simulink model "project1_Harrington_and_Mckeon"  (R2025a)
settings: Solver=VariableStepAuto  StartTime=0.0  StopTime=30  RelTol=1e-3
model workspace (MAT data in the model file):
  A = 972
  M1 = 300
  M2 = 75
  g = 1.62
  k = 9000
  mu = 0.2
undefined symbols (not defined in the file): pulse
libraries: simulink x1
settings Model: Creator=brendan  LastModifiedBy=brendanharrington

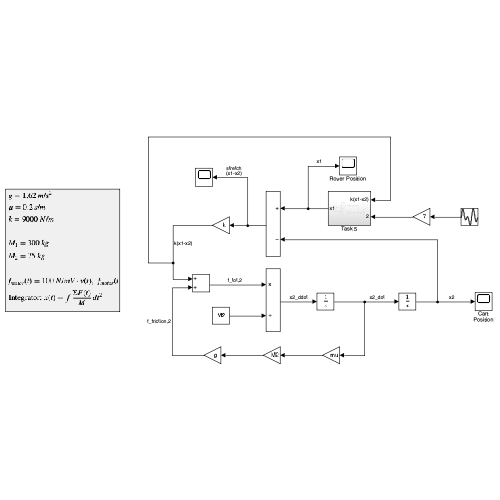
[thumbnail: Simulink's stored preview of the top-level diagram]
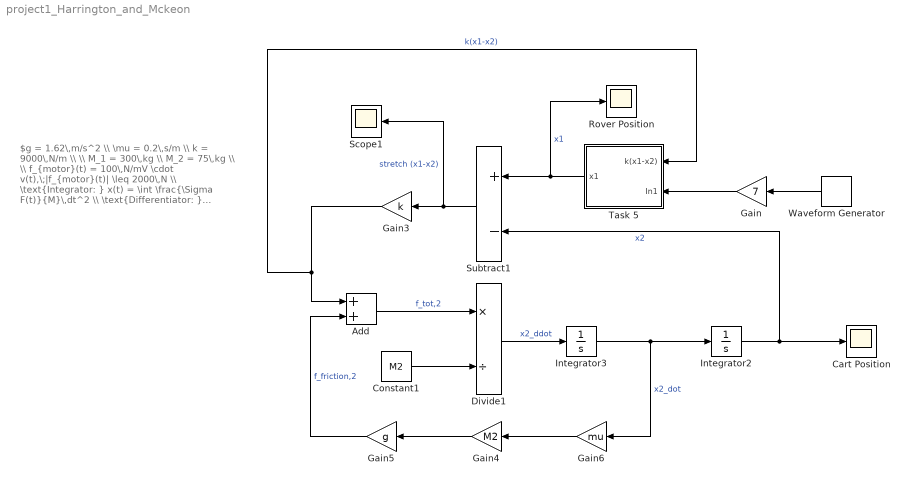
== system project1_Harrington_and_Mckeon ==
  note: $g = 1.62\,m/s^2 \\ \mu = 0.2\,s/m \\ k = 9000\,N/m \\ \\ M_1 = 300\,kg \\ M_2 = 75\,kg \\ \\ f_{motor}(t) = 100\,N/mV \cdot v(t),\;|f_{motor}(t)| \leq 2000\,N \\ \text{Integrator: } x(t) = \int \frac{\Sigma F(t)}{M}\,dt^2 \\ \text{Differentiator: } f_{friction}(t) = -\mu M g\,\dot{x}(t) \\ \\ \frac{X_1(s)}{F_{motor}(s)} = \frac{1}{M_1(s^2+\mu g s)}$
  Add : Sum
  Cart Position : Scope
      settings: ActiveDisplayYMinimum=-12.04250247875151  ActiveDisplayYMaximum=108.38252230876363  DataLoggingVariableName=ScopeData4
  Constant1 : Constant  Value=M2
  Divide1 : Product  Inputs=*/
  Gain : Gain  Gain=7
  Gain3 : Gain  Gain=k
  Gain4 : Gain  Gain=M2
  Gain5 : Gain  Gain=g
  Gain6 : Gain  Gain=mu
  Integrator2 : Integrator
  Integrator3 : Integrator
  Rover Position : Scope
      settings: ActiveDisplayYMinimum=-34.346909890801307  ActiveDisplayYMaximum=309.12218901721184
  Scope1 : Scope
      settings: ActiveDisplayYMinimum=-1  ActiveDisplayYMaximum=1
  Subtract1 : Sum  Inputs=+-
  Task 5 : Subsystem
  Waveform Generator : simulink/Sources/Waveform Generator  OutMin=[]  OutMax=[]  OutDataTypeStr=double  SelectedSignal=1  Signals=pulse(1,0,10)  BlockNames=MultiportSwitch_55af036a47ab4e6  SampleTime=0.1
  wires:
  Gain5/1 -> Add/2  "f_friction,2"
  Constant1/1 -> Divide1/2
  Gain6/1 -> Gain4/1
  Integrator2/1 -> Cart Position/1, Subtract1/2  "x2"
  Gain4/1 -> Gain5/1
  Gain3/1 -> Task 5/1(k(x1-x2)), Add/1  "k(x1-x2)"
  Integrator3/1 -> Gain6/1, Integrator2/1  "x2_dot"
  Divide1/1 -> Integrator3/1  "x2_ddot"
  Task 5/1(x1) -> Rover Position/1, Subtract1/1  "x1"
  Subtract1/1 -> Gain3/1, Scope1/1  "stretch (x1-x2)"
  Add/1 -> Divide1/1  "f_tot,2"
  Waveform Generator/1 -> Gain/1
  Gain/1 -> Task 5/2(In1)

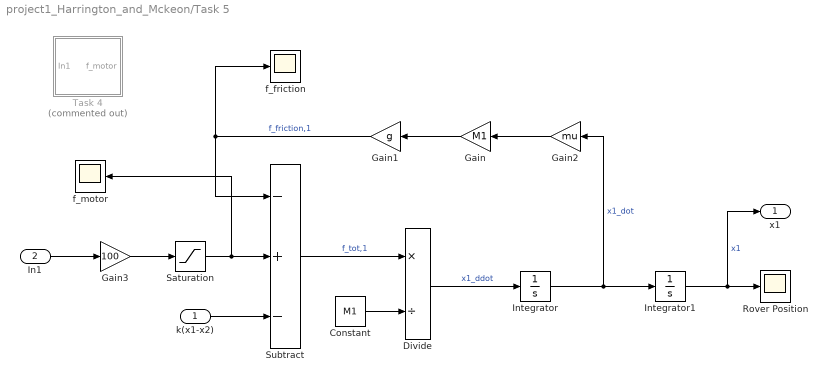
== system project1_Harrington_and_Mckeon/Task 5 ==
  k(x1-x2) : Inport
  In1 : Inport  Port=2
  Constant : Constant  Value=M1
  Divide : Product  Inputs=*/
  Gain : Gain  Gain=M1
  Gain1 : Gain  Gain=g
  Gain2 : Gain  Gain=mu
  Gain3 : Gain  Gain=100
  Integrator : Integrator
  Integrator1 : Integrator
  Rover Position : Scope
      settings: ActiveDisplayYMinimum=-12.494314268256833  ActiveDisplayYMaximum=112.44882841431152
  Saturation : Saturate  UpperLimit=2000  LowerLimit=-2000
  Subtract : Sum  Inputs=-+-
  Task 4 : Subsystem  Commented=on
  f_friction : Scope
      settings: ActiveDisplayYMinimum=-1  ActiveDisplayYMaximum=1  DataLoggingVariableName=ScopeData2
  f_motor : Scope
      settings: ActiveDisplayYMinimum=-1  ActiveDisplayYMaximum=1
  x1 : Outport
  wires:
  Integrator/1 -> Integrator1/1, Gain2/1  "x1_dot"
  Constant/1 -> Divide/2
  Gain1/1 -> Subtract/1, f_friction/1  "f_friction,1"
  Divide/1 -> Integrator/1  "x1_ddot"
  Gain2/1 -> Gain/1
  Gain/1 -> Gain1/1
  Subtract/1 -> Divide/1  "f_tot,1"
  Integrator1/1 -> x1/1, Rover Position/1  "x1"
  k(x1-x2)/1 -> Subtract/3
  In1/1 -> Gain3/1
  Gain3/1 -> Saturation/1
  Saturation/1 -> f_motor/1, Subtract/2

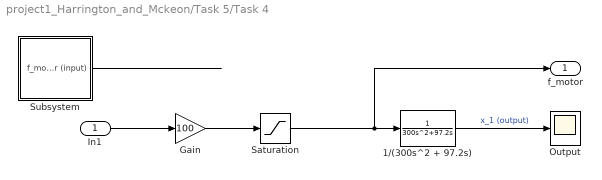
== system project1_Harrington_and_Mckeon/Task 5/Task 4 ==
  In1 : Inport
  1/(300s^2 + 97.2s) : TransferFcn  Denominator=[300 97.2 0]
  Gain : Gain  Gain=100
  Output : Scope
      settings: ActiveDisplayYMinimum=-27.497526566550121  ActiveDisplayYMaximum=129.99510038360791  DataLoggingVariableName=ScopeData3
  Saturation : Saturate  UpperLimit=2000  LowerLimit=-2000
  Subsystem : Subsystem
  f_motor : Outport
  wires:
  1/(300s^2 + 97.2s)/1 -> Output/1  "x_1 (output)"
  Saturation/1 -> f_motor/1, 1/(300s^2 + 97.2s)/1
  Subsystem/1(f_motor (input)) -> ?
  In1/1 -> Gain/1
  Gain/1 -> Saturation/1

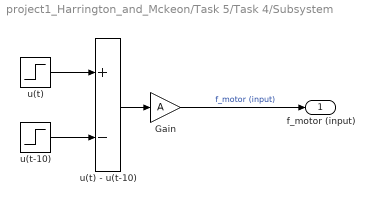
== system project1_Harrington_and_Mckeon/Task 5/Task 4/Subsystem ==
  Gain : Gain  Gain=A
  u(t) : Step  Time=0  SampleTime=0
  u(t) - u(t-10) : Sum  Inputs=+-
  u(t-10) : Step  Time=10  SampleTime=0
  f_motor (input) : Outport
  wires:
  Gain/1 -> f_motor (input)/1  "f_motor (input)"
  u(t)/1 -> u(t) - u(t-10)/1
  u(t-10)/1 -> u(t) - u(t-10)/2
  u(t) - u(t-10)/1 -> Gain/1
